simulink model "Model_with_decision"  (R2022a)
settings: Solver=VariableStepAuto  StartTime=0.0  StopTime=1000000  RelTol=1e-3
undefined symbols (not defined in the file): Coefficient_value, Enable_X, Enable_Y, N, s1, s10, s11, s12, s13, s14, s15, s16, s17, s18, s19, s2, s20, s21, s22, s23, s24, s25, s26, s27, s28, s29, s3, s30, s4, s5, s6, s7, s8, s9
libraries: simulink x35
(part 3 of 5)

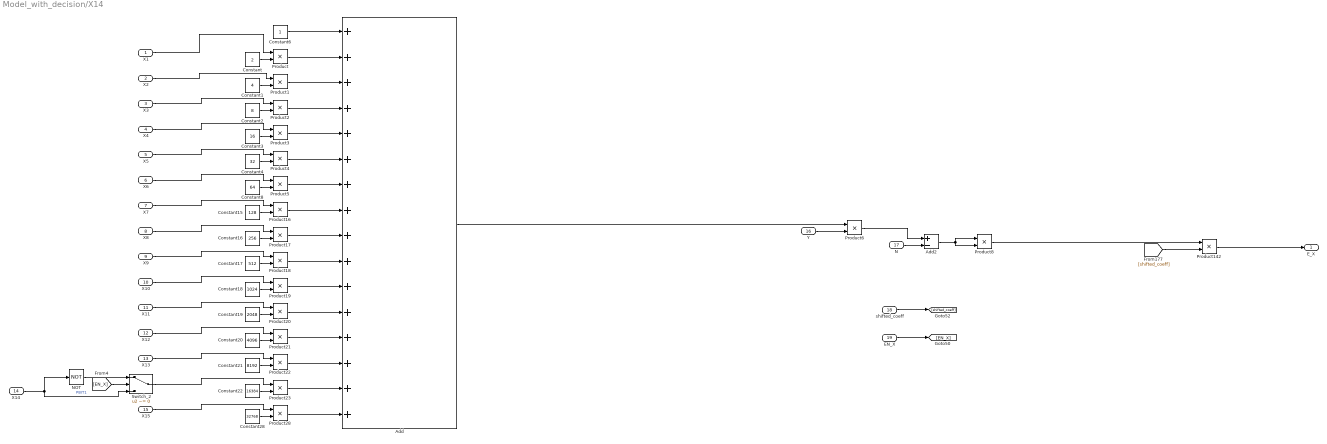
== system Model_with_decision/X14 ==
  X1 : Inport  OutDataTypeStr=fixdt(0,1,0)  LockScale=on
  X2 : Inport  Port=2  OutDataTypeStr=fixdt(0,1,0)  LockScale=on
  X3 : Inport  Port=3  OutDataTypeStr=fixdt(0,1,0)  LockScale=on
  X4 : Inport  Port=4  OutDataTypeStr=fixdt(0,1,0)  LockScale=on
  X5 : Inport  Port=5  OutDataTypeStr=fixdt(0,1,0)  LockScale=on
  X6 : Inport  Port=6  OutDataTypeStr=fixdt(0,1,0)  LockScale=on
  X7 : Inport  Port=7  OutDataTypeStr=fixdt(0,1,0)  LockScale=on
  X8 : Inport  Port=8  OutDataTypeStr=fixdt(0,1,0)  LockScale=on
  X9 : Inport  Port=9  OutDataTypeStr=fixdt(0,1,0)  LockScale=on
  X10 : Inport  Port=10  OutDataTypeStr=fixdt(0,1,0)  LockScale=on
  X11 : Inport  Port=11  OutDataTypeStr=fixdt(0,1,0)  LockScale=on
  X12 : Inport  Port=12  OutDataTypeStr=fixdt(0,1,0)  LockScale=on
  X13 : Inport  Port=13  OutDataTypeStr=fixdt(0,1,0)  LockScale=on
  X14 : Inport  Port=14  OutDataTypeStr=fixdt(0,1,0)  LockScale=on
  X15 : Inport  Port=15  OutDataTypeStr=fixdt(0,1,0)  LockScale=on
  Y : Inport  Port=16  LockScale=on
  N : Inport  Port=17  LockScale=on
  shifted_coeff : Inport  Port=18  LockScale=on
  EN_X : Inport  Port=19  OutDataTypeStr=fixdt(0,1,0)  LockScale=on
  Add : Sum  Inputs=++++++++++++++++
  Add2 : Sum  Inputs=+-
  Constant : Constant  Value=2
  Constant1 : Constant  Value=4
  Constant15 : Constant  Value=128
  Constant16 : Constant  Value=256
  Constant17 : Constant  Value=512
  Constant18 : Constant  Value=1024
  Constant19 : Constant  Value=2048
  Constant2 : Constant  Value=8
  Constant20 : Constant  Value=4096
  Constant21 : Constant  Value=8192
  Constant22 : Constant  Value=16384
  Constant28 : Constant  Value=32768
  Constant3 : Constant  Value=16
  Constant4 : Constant  Value=32
  Constant6 : Constant
  Constant8 : Constant  Value=64
  NOT : Logic  Operator=NOT  IconShape=distinctive  AllPortsSameDT=off  OutDataTypeStr=boolean
  Product{,1..6,8,16..23,28,142} (18 alike) : Product
  Switch_2 : Switch  Criteria=u2 ~= 0  OutDataTypeStr=fixdt(0,1,0)  SaturateOnIntegerOverflow=off  InputSameDT=off
  E_X : Outport  LockScale=on
  wires:
  Y/1 -> Product6/2
  N/1 -> Add2/2
  Product8/1 -> Product142/1
  Product6/1 -> Add2/1
  [shifted_coeff] -> Product142/2
  Product142/1 -> E_X/1
  shifted_coeff/1 -> [shifted_coeff]
  EN_X/1 -> [EN_X]
  X13/1 -> Product22/1
  NOT/1 -> Switch_2/1
  X14/1 -> NOT/1, Switch_2/3  "PBIT1"
  [EN_X] -> Switch_2/2
  Constant22/1 -> Product23/2
  Constant21/1 -> Product22/2
  Product23/1 -> Add/15
  Product22/1 -> Add/14
  Product28/1 -> Add/16
  Constant28/1 -> Product28/2
  X15/1 -> Product28/1
  Switch_2/1 -> Product23/1
  Product17/1 -> Add/9
  X12/1 -> Product21/1
  Product21/1 -> Add/13
  Constant17/1 -> Product18/2
  X9/1 -> Product18/1
  Product16/1 -> Add/8
  Constant19/1 -> Product20/2
  X7/1 -> Product16/1
  X10/1 -> Product19/1
  X8/1 -> Product17/1
  Product20/1 -> Add/12
  X11/1 -> Product20/1
  Constant16/1 -> Product17/2
  Constant15/1 -> Product16/2
  Product18/1 -> Add/10
  Constant18/1 -> Product19/2
  Constant20/1 -> Product21/2
  Product19/1 -> Add/11
  Constant3/1 -> Product3/2
  X5/1 -> Product4/1
  Product5/1 -> Add/7
  X4/1 -> Product3/1
  Product3/1 -> Add/5
  X6/1 -> Product5/1
  Constant8/1 -> Product5/2
  Constant4/1 -> Product4/2
  Product4/1 -> Add/6
  Add2/1 -> Product8/1, Product8/2
  Add/1 -> Product6/1
  Product2/1 -> Add/4
  Product1/1 -> Add/3
  Product/1 -> Add/2
  Constant6/1 -> Add/1
  X3/1 -> Product2/1
  Constant2/1 -> Product2/2
  X2/1 -> Product1/1
  Constant1/1 -> Product1/2
  X1/1 -> Product/1
  Constant/1 -> Product/2

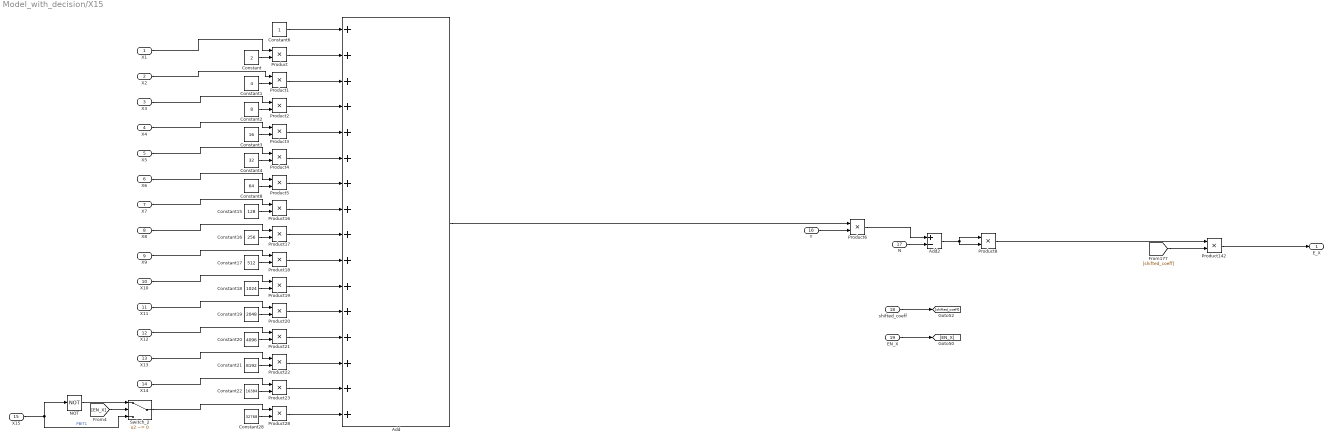
== system Model_with_decision/X15 ==
  X1 : Inport  OutDataTypeStr=fixdt(0,1,0)  LockScale=on
  X2 : Inport  Port=2  OutDataTypeStr=fixdt(0,1,0)  LockScale=on
  X3 : Inport  Port=3  OutDataTypeStr=fixdt(0,1,0)  LockScale=on
  X4 : Inport  Port=4  OutDataTypeStr=fixdt(0,1,0)  LockScale=on
  X5 : Inport  Port=5  OutDataTypeStr=fixdt(0,1,0)  LockScale=on
  X6 : Inport  Port=6  OutDataTypeStr=fixdt(0,1,0)  LockScale=on
  X7 : Inport  Port=7  OutDataTypeStr=fixdt(0,1,0)  LockScale=on
  X8 : Inport  Port=8  OutDataTypeStr=fixdt(0,1,0)  LockScale=on
  X9 : Inport  Port=9  OutDataTypeStr=fixdt(0,1,0)  LockScale=on
  X10 : Inport  Port=10  OutDataTypeStr=fixdt(0,1,0)  LockScale=on
  X11 : Inport  Port=11  OutDataTypeStr=fixdt(0,1,0)  LockScale=on
  X12 : Inport  Port=12  OutDataTypeStr=fixdt(0,1,0)  LockScale=on
  X13 : Inport  Port=13  OutDataTypeStr=fixdt(0,1,0)  LockScale=on
  X14 : Inport  Port=14  OutDataTypeStr=fixdt(0,1,0)  LockScale=on
  X15 : Inport  Port=15  OutDataTypeStr=fixdt(0,1,0)  LockScale=on
  Y : Inport  Port=16  LockScale=on
  N : Inport  Port=17  LockScale=on
  shifted_coeff : Inport  Port=18  LockScale=on
  EN_X : Inport  Port=19  OutDataTypeStr=fixdt(0,1,0)  LockScale=on
  Add : Sum  Inputs=++++++++++++++++
  Add2 : Sum  Inputs=+-
  Constant : Constant  Value=2
  Constant1 : Constant  Value=4
  Constant15 : Constant  Value=128
  Constant16 : Constant  Value=256
  Constant17 : Constant  Value=512
  Constant18 : Constant  Value=1024
  Constant19 : Constant  Value=2048
  Constant2 : Constant  Value=8
  Constant20 : Constant  Value=4096
  Constant21 : Constant  Value=8192
  Constant22 : Constant  Value=16384
  Constant28 : Constant  Value=32768
  Constant3 : Constant  Value=16
  Constant4 : Constant  Value=32
  Constant6 : Constant
  Constant8 : Constant  Value=64
  NOT : Logic  Operator=NOT  IconShape=distinctive  AllPortsSameDT=off  OutDataTypeStr=boolean
  Product{,1..6,8,16..23,28,142} (18 alike) : Product
  Switch_2 : Switch  Criteria=u2 ~= 0  OutDataTypeStr=fixdt(0,1,0)  SaturateOnIntegerOverflow=off  InputSameDT=off
  E_X : Outport  LockScale=on
  wires:
  Constant/1 -> Product/2
  X1/1 -> Product/1
  Constant1/1 -> Product1/2
  X2/1 -> Product1/1
  Constant2/1 -> Product2/2
  X3/1 -> Product2/1
  Constant6/1 -> Add/1
  Product/1 -> Add/2
  Product1/1 -> Add/3
  Product2/1 -> Add/4
  Add/1 -> Product6/1
  Add2/1 -> Product8/2, Product8/1
  Product4/1 -> Add/6
  Constant4/1 -> Product4/2
  Constant8/1 -> Product5/2
  X6/1 -> Product5/1
  Product3/1 -> Add/5
  X4/1 -> Product3/1
  Product5/1 -> Add/7
  X5/1 -> Product4/1
  Constant3/1 -> Product3/2
  Product19/1 -> Add/11
  Constant20/1 -> Product21/2
  Constant18/1 -> Product19/2
  Product18/1 -> Add/10
  Constant15/1 -> Product16/2
  Constant16/1 -> Product17/2
  X11/1 -> Product20/1
  Product20/1 -> Add/12
  X8/1 -> Product17/1
  X10/1 -> Product19/1
  X7/1 -> Product16/1
  Constant19/1 -> Product20/2
  Product16/1 -> Add/8
  X9/1 -> Product18/1
  Constant17/1 -> Product18/2
  Product21/1 -> Add/13
  X12/1 -> Product21/1
  Product17/1 -> Add/9
  X14/1 -> Product23/1
  Switch_2/1 -> Product28/1
  Constant28/1 -> Product28/2
  Product28/1 -> Add/16
  Product22/1 -> Add/14
  Product23/1 -> Add/15
  Constant21/1 -> Product22/2
  Constant22/1 -> Product23/2
  [EN_X] -> Switch_2/2
  X15/1 -> Switch_2/3, NOT/1  "PBIT1"
  NOT/1 -> Switch_2/1
  X13/1 -> Product22/1
  EN_X/1 -> [EN_X]
  shifted_coeff/1 -> [shifted_coeff]
  Product142/1 -> E_X/1
  [shifted_coeff] -> Product142/2
  Product6/1 -> Add2/1
  Product8/1 -> Product142/1
  N/1 -> Add2/2
  Y/1 -> Product6/2

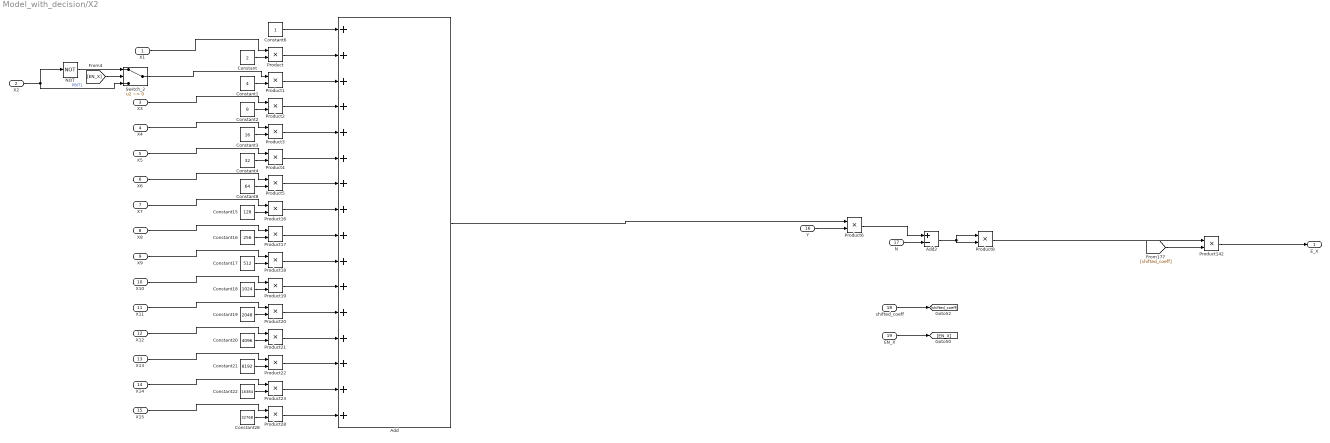
== system Model_with_decision/X2 ==
  X1 : Inport  OutDataTypeStr=fixdt(0,1,0)  LockScale=on
  X2 : Inport  Port=2  OutDataTypeStr=fixdt(0,1,0)  LockScale=on
  X3 : Inport  Port=3  OutDataTypeStr=fixdt(0,1,0)  LockScale=on
  X4 : Inport  Port=4  OutDataTypeStr=fixdt(0,1,0)  LockScale=on
  X5 : Inport  Port=5  OutDataTypeStr=fixdt(0,1,0)  LockScale=on
  X6 : Inport  Port=6  OutDataTypeStr=fixdt(0,1,0)  LockScale=on
  X7 : Inport  Port=7  OutDataTypeStr=fixdt(0,1,0)  LockScale=on
  X8 : Inport  Port=8  OutDataTypeStr=fixdt(0,1,0)  LockScale=on
  X9 : Inport  Port=9  OutDataTypeStr=fixdt(0,1,0)  LockScale=on
  X10 : Inport  Port=10  OutDataTypeStr=fixdt(0,1,0)  LockScale=on
  X11 : Inport  Port=11  OutDataTypeStr=fixdt(0,1,0)  LockScale=on
  X12 : Inport  Port=12  OutDataTypeStr=fixdt(0,1,0)  LockScale=on
  X13 : Inport  Port=13  OutDataTypeStr=fixdt(0,1,0)  LockScale=on
  X14 : Inport  Port=14  OutDataTypeStr=fixdt(0,1,0)  LockScale=on
  X15 : Inport  Port=15  OutDataTypeStr=fixdt(0,1,0)  LockScale=on
  Y : Inport  Port=16  LockScale=on
  N : Inport  Port=17  LockScale=on
  shifted_coeff : Inport  Port=18  LockScale=on
  EN_X : Inport  Port=19  OutDataTypeStr=fixdt(0,1,0)  LockScale=on
  Add : Sum  Inputs=++++++++++++++++
  Add2 : Sum  Inputs=+-
  Constant : Constant  Value=2
  Constant1 : Constant  Value=4
  Constant15 : Constant  Value=128
  Constant16 : Constant  Value=256
  Constant17 : Constant  Value=512
  Constant18 : Constant  Value=1024
  Constant19 : Constant  Value=2048
  Constant2 : Constant  Value=8
  Constant20 : Constant  Value=4096
  Constant21 : Constant  Value=8192
  Constant22 : Constant  Value=16384
  Constant28 : Constant  Value=32768
  Constant3 : Constant  Value=16
  Constant4 : Constant  Value=32
  Constant6 : Constant
  Constant8 : Constant  Value=64
  NOT : Logic  Operator=NOT  IconShape=distinctive  AllPortsSameDT=off  OutDataTypeStr=boolean
  Product{,1..6,8,16..23,28,142} (18 alike) : Product
  Switch_2 : Switch  Criteria=u2 ~= 0  OutDataTypeStr=fixdt(0,1,0)  SaturateOnIntegerOverflow=off  InputSameDT=off
  E_X : Outport  LockScale=on
  wires:
  Y/1 -> Product6/2
  N/1 -> Add2/2
  Product8/1 -> Product142/1
  Product6/1 -> Add2/1
  [shifted_coeff] -> Product142/2
  Product142/1 -> E_X/1
  shifted_coeff/1 -> [shifted_coeff]
  EN_X/1 -> [EN_X]
  X13/1 -> Product22/1
  NOT/1 -> Switch_2/1
  X2/1 -> Switch_2/3, NOT/1  "PBIT1"
  [EN_X] -> Switch_2/2
  Constant22/1 -> Product23/2
  Constant21/1 -> Product22/2
  Product23/1 -> Add/15
  Product22/1 -> Add/14
  Product28/1 -> Add/16
  Constant28/1 -> Product28/2
  X15/1 -> Product28/1
  X14/1 -> Product23/1
  Product17/1 -> Add/9
  X12/1 -> Product21/1
  Product21/1 -> Add/13
  Constant17/1 -> Product18/2
  X9/1 -> Product18/1
  Product16/1 -> Add/8
  Constant19/1 -> Product20/2
  X7/1 -> Product16/1
  X10/1 -> Product19/1
  X8/1 -> Product17/1
  Product20/1 -> Add/12
  X11/1 -> Product20/1
  Constant16/1 -> Product17/2
  Constant15/1 -> Product16/2
  Product18/1 -> Add/10
  Constant18/1 -> Product19/2
  Constant20/1 -> Product21/2
  Product19/1 -> Add/11
  Constant3/1 -> Product3/2
  X5/1 -> Product4/1
  Product5/1 -> Add/7
  X4/1 -> Product3/1
  Product3/1 -> Add/5
  X6/1 -> Product5/1
  Constant8/1 -> Product5/2
  Constant4/1 -> Product4/2
  Product4/1 -> Add/6
  Add2/1 -> Product8/1, Product8/2
  Add/1 -> Product6/1
  Product2/1 -> Add/4
  Product1/1 -> Add/3
  Product/1 -> Add/2
  Constant6/1 -> Add/1
  X3/1 -> Product2/1
  Constant2/1 -> Product2/2
  Switch_2/1 -> Product1/1
  Constant1/1 -> Product1/2
  X1/1 -> Product/1
  Constant/1 -> Product/2

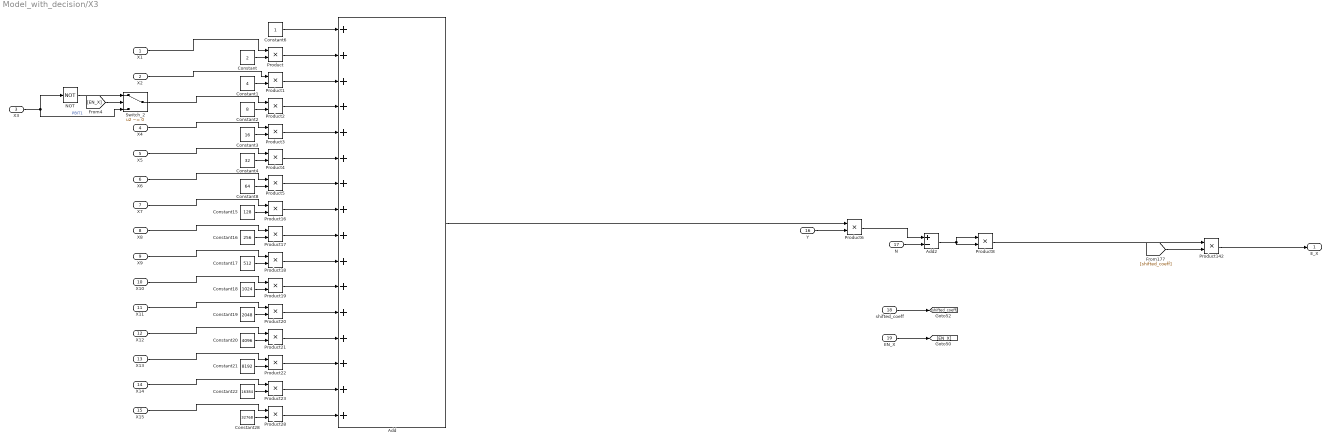
== system Model_with_decision/X3 ==
  X1 : Inport  OutDataTypeStr=fixdt(0,1,0)  LockScale=on
  X2 : Inport  Port=2  OutDataTypeStr=fixdt(0,1,0)  LockScale=on
  X3 : Inport  Port=3  OutDataTypeStr=fixdt(0,1,0)  LockScale=on
  X4 : Inport  Port=4  OutDataTypeStr=fixdt(0,1,0)  LockScale=on
  X5 : Inport  Port=5  OutDataTypeStr=fixdt(0,1,0)  LockScale=on
  X6 : Inport  Port=6  OutDataTypeStr=fixdt(0,1,0)  LockScale=on
  X7 : Inport  Port=7  OutDataTypeStr=fixdt(0,1,0)  LockScale=on
  X8 : Inport  Port=8  OutDataTypeStr=fixdt(0,1,0)  LockScale=on
  X9 : Inport  Port=9  OutDataTypeStr=fixdt(0,1,0)  LockScale=on
  X10 : Inport  Port=10  OutDataTypeStr=fixdt(0,1,0)  LockScale=on
  X11 : Inport  Port=11  OutDataTypeStr=fixdt(0,1,0)  LockScale=on
  X12 : Inport  Port=12  OutDataTypeStr=fixdt(0,1,0)  LockScale=on
  X13 : Inport  Port=13  OutDataTypeStr=fixdt(0,1,0)  LockScale=on
  X14 : Inport  Port=14  OutDataTypeStr=fixdt(0,1,0)  LockScale=on
  X15 : Inport  Port=15  OutDataTypeStr=fixdt(0,1,0)  LockScale=on
  Y : Inport  Port=16  LockScale=on
  N : Inport  Port=17  LockScale=on
  shifted_coeff : Inport  Port=18  LockScale=on
  EN_X : Inport  Port=19  OutDataTypeStr=fixdt(0,1,0)  LockScale=on
  Add : Sum  Inputs=++++++++++++++++
  Add2 : Sum  Inputs=+-
  Constant : Constant  Value=2
  Constant1 : Constant  Value=4
  Constant15 : Constant  Value=128
  Constant16 : Constant  Value=256
  Constant17 : Constant  Value=512
  Constant18 : Constant  Value=1024
  Constant19 : Constant  Value=2048
  Constant2 : Constant  Value=8
  Constant20 : Constant  Value=4096
  Constant21 : Constant  Value=8192
  Constant22 : Constant  Value=16384
  Constant28 : Constant  Value=32768
  Constant3 : Constant  Value=16
  Constant4 : Constant  Value=32
  Constant6 : Constant
  Constant8 : Constant  Value=64
  NOT : Logic  Operator=NOT  IconShape=distinctive  AllPortsSameDT=off  OutDataTypeStr=boolean
  Product{,1..6,8,16..23,28,142} (18 alike) : Product
  Switch_2 : Switch  Criteria=u2 ~= 0  OutDataTypeStr=fixdt(0,1,0)  SaturateOnIntegerOverflow=off  InputSameDT=off
  E_X : Outport  LockScale=on
  wires:
  Y/1 -> Product6/2
  N/1 -> Add2/2
  Product8/1 -> Product142/1
  Product6/1 -> Add2/1
  [shifted_coeff] -> Product142/2
  Product142/1 -> E_X/1
  shifted_coeff/1 -> [shifted_coeff]
  EN_X/1 -> [EN_X]
  X13/1 -> Product22/1
  NOT/1 -> Switch_2/1
  X3/1 -> Switch_2/3, NOT/1  "PBIT1"
  [EN_X] -> Switch_2/2
  Constant22/1 -> Product23/2
  Constant21/1 -> Product22/2
  Product23/1 -> Add/15
  Product22/1 -> Add/14
  Product28/1 -> Add/16
  Constant28/1 -> Product28/2
  X15/1 -> Product28/1
  X14/1 -> Product23/1
  Product17/1 -> Add/9
  X12/1 -> Product21/1
  Product21/1 -> Add/13
  Constant17/1 -> Product18/2
  X9/1 -> Product18/1
  Product16/1 -> Add/8
  Constant19/1 -> Product20/2
  X7/1 -> Product16/1
  X10/1 -> Product19/1
  X8/1 -> Product17/1
  Product20/1 -> Add/12
  X11/1 -> Product20/1
  Constant16/1 -> Product17/2
  Constant15/1 -> Product16/2
  Product18/1 -> Add/10
  Constant18/1 -> Product19/2
  Constant20/1 -> Product21/2
  Product19/1 -> Add/11
  Constant3/1 -> Product3/2
  X5/1 -> Product4/1
  Product5/1 -> Add/7
  X4/1 -> Product3/1
  Product3/1 -> Add/5
  X6/1 -> Product5/1
  Constant8/1 -> Product5/2
  Constant4/1 -> Product4/2
  Product4/1 -> Add/6
  Add2/1 -> Product8/1, Product8/2
  Add/1 -> Product6/1
  Product2/1 -> Add/4
  Product1/1 -> Add/3
  Product/1 -> Add/2
  Constant6/1 -> Add/1
  Switch_2/1 -> Product2/1
  Constant2/1 -> Product2/2
  X2/1 -> Product1/1
  Constant1/1 -> Product1/2
  X1/1 -> Product/1
  Constant/1 -> Product/2

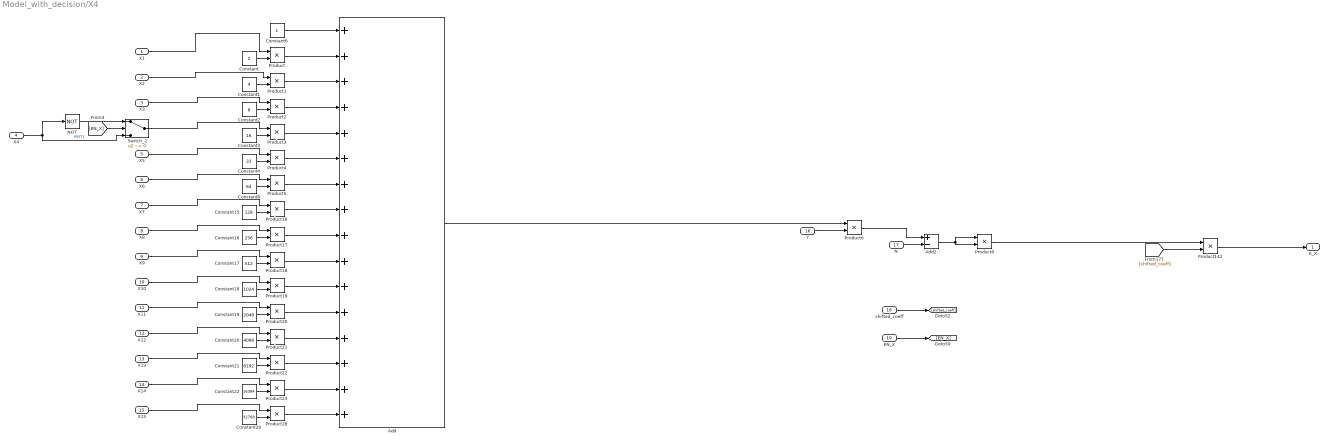
== system Model_with_decision/X4 ==
  X1 : Inport  OutDataTypeStr=fixdt(0,1,0)  LockScale=on
  X2 : Inport  Port=2  OutDataTypeStr=fixdt(0,1,0)  LockScale=on
  X3 : Inport  Port=3  OutDataTypeStr=fixdt(0,1,0)  LockScale=on
  X4 : Inport  Port=4  OutDataTypeStr=fixdt(0,1,0)  LockScale=on
  X5 : Inport  Port=5  OutDataTypeStr=fixdt(0,1,0)  LockScale=on
  X6 : Inport  Port=6  OutDataTypeStr=fixdt(0,1,0)  LockScale=on
  X7 : Inport  Port=7  OutDataTypeStr=fixdt(0,1,0)  LockScale=on
  X8 : Inport  Port=8  OutDataTypeStr=fixdt(0,1,0)  LockScale=on
  X9 : Inport  Port=9  OutDataTypeStr=fixdt(0,1,0)  LockScale=on
  X10 : Inport  Port=10  OutDataTypeStr=fixdt(0,1,0)  LockScale=on
  X11 : Inport  Port=11  OutDataTypeStr=fixdt(0,1,0)  LockScale=on
  X12 : Inport  Port=12  OutDataTypeStr=fixdt(0,1,0)  LockScale=on
  X13 : Inport  Port=13  OutDataTypeStr=fixdt(0,1,0)  LockScale=on
  X14 : Inport  Port=14  OutDataTypeStr=fixdt(0,1,0)  LockScale=on
  X15 : Inport  Port=15  OutDataTypeStr=fixdt(0,1,0)  LockScale=on
  Y : Inport  Port=16  LockScale=on
  N : Inport  Port=17  LockScale=on
  shifted_coeff : Inport  Port=18  LockScale=on
  EN_X : Inport  Port=19  OutDataTypeStr=fixdt(0,1,0)  LockScale=on
  Add : Sum  Inputs=++++++++++++++++
  Add2 : Sum  Inputs=+-
  Constant : Constant  Value=2
  Constant1 : Constant  Value=4
  Constant15 : Constant  Value=128
  Constant16 : Constant  Value=256
  Constant17 : Constant  Value=512
  Constant18 : Constant  Value=1024
  Constant19 : Constant  Value=2048
  Constant2 : Constant  Value=8
  Constant20 : Constant  Value=4096
  Constant21 : Constant  Value=8192
  Constant22 : Constant  Value=16384
  Constant28 : Constant  Value=32768
  Constant3 : Constant  Value=16
  Constant4 : Constant  Value=32
  Constant6 : Constant
  Constant8 : Constant  Value=64
  NOT : Logic  Operator=NOT  IconShape=distinctive  AllPortsSameDT=off  OutDataTypeStr=boolean
  Product{,1..6,8,16..23,28,142} (18 alike) : Product
  Switch_2 : Switch  Criteria=u2 ~= 0  OutDataTypeStr=fixdt(0,1,0)  SaturateOnIntegerOverflow=off  InputSameDT=off
  E_X : Outport  LockScale=on
  wires:
  Constant/1 -> Product/2
  X1/1 -> Product/1
  Constant1/1 -> Product1/2
  X2/1 -> Product1/1
  Constant2/1 -> Product2/2
  X3/1 -> Product2/1
  Constant6/1 -> Add/1
  Product/1 -> Add/2
  Product1/1 -> Add/3
  Product2/1 -> Add/4
  Add/1 -> Product6/1
  Add2/1 -> Product8/2, Product8/1
  Product4/1 -> Add/6
  Constant4/1 -> Product4/2
  Constant8/1 -> Product5/2
  X6/1 -> Product5/1
  Product3/1 -> Add/5
  Switch_2/1 -> Product3/1
  Product5/1 -> Add/7
  X5/1 -> Product4/1
  Constant3/1 -> Product3/2
  Product19/1 -> Add/11
  Constant20/1 -> Product21/2
  Constant18/1 -> Product19/2
  Product18/1 -> Add/10
  Constant15/1 -> Product16/2
  Constant16/1 -> Product17/2
  X11/1 -> Product20/1
  Product20/1 -> Add/12
  X8/1 -> Product17/1
  X10/1 -> Product19/1
  X7/1 -> Product16/1
  Constant19/1 -> Product20/2
  Product16/1 -> Add/8
  X9/1 -> Product18/1
  Constant17/1 -> Product18/2
  Product21/1 -> Add/13
  X12/1 -> Product21/1
  Product17/1 -> Add/9
  X14/1 -> Product23/1
  X15/1 -> Product28/1
  Constant28/1 -> Product28/2
  Product28/1 -> Add/16
  Product22/1 -> Add/14
  Product23/1 -> Add/15
  Constant21/1 -> Product22/2
  Constant22/1 -> Product23/2
  [EN_X] -> Switch_2/2
  X4/1 -> NOT/1, Switch_2/3  "PBIT1"
  NOT/1 -> Switch_2/1
  X13/1 -> Product22/1
  EN_X/1 -> [EN_X]
  shifted_coeff/1 -> [shifted_coeff]
  Product142/1 -> E_X/1
  [shifted_coeff] -> Product142/2
  Product6/1 -> Add2/1
  Product8/1 -> Product142/1
  N/1 -> Add2/2
  Y/1 -> Product6/2

== system Model_with_decision/X5 ==
  X1 : Inport  OutDataTypeStr=fixdt(0,1,0)  LockScale=on
  X2 : Inport  Port=2  OutDataTypeStr=fixdt(0,1,0)  LockScale=on
  X3 : Inport  Port=3  OutDataTypeStr=fixdt(0,1,0)  LockScale=on
  X4 : Inport  Port=4  OutDataTypeStr=fixdt(0,1,0)  LockScale=on
  X5 : Inport  Port=5  OutDataTypeStr=fixdt(0,1,0)  LockScale=on
  X6 : Inport  Port=6  OutDataTypeStr=fixdt(0,1,0)  LockScale=on
  X7 : Inport  Port=7  OutDataTypeStr=fixdt(0,1,0)  LockScale=on
  X8 : Inport  Port=8  OutDataTypeStr=fixdt(0,1,0)  LockScale=on
  X9 : Inport  Port=9  OutDataTypeStr=fixdt(0,1,0)  LockScale=on
  X10 : Inport  Port=10  OutDataTypeStr=fixdt(0,1,0)  LockScale=on
  X11 : Inport  Port=11  OutDataTypeStr=fixdt(0,1,0)  LockScale=on
  X12 : Inport  Port=12  OutDataTypeStr=fixdt(0,1,0)  LockScale=on
  X13 : Inport  Port=13  OutDataTypeStr=fixdt(0,1,0)  LockScale=on
  X14 : Inport  Port=14  OutDataTypeStr=fixdt(0,1,0)  LockScale=on
  X15 : Inport  Port=15  OutDataTypeStr=fixdt(0,1,0)  LockScale=on
  Y : Inport  Port=16  LockScale=on
  N : Inport  Port=17  LockScale=on
  shifted_coeff : Inport  Port=18  LockScale=on
  EN_X : Inport  Port=19  OutDataTypeStr=fixdt(0,1,0)  LockScale=on
  Add : Sum  Inputs=++++++++++++++++
  Add2 : Sum  Inputs=+-
  Constant : Constant  Value=2
  Constant1 : Constant  Value=4
  Constant15 : Constant  Value=128
  Constant16 : Constant  Value=256
  Constant17 : Constant  Value=512
  Constant18 : Constant  Value=1024
  Constant19 : Constant  Value=2048
  Constant2 : Constant  Value=8
  Constant20 : Constant  Value=4096
  Constant21 : Constant  Value=8192
  Constant22 : Constant  Value=16384
  Constant28 : Constant  Value=32768
  Constant3 : Constant  Value=16
  Constant4 : Constant  Value=32
  Constant6 : Constant
  Constant8 : Constant  Value=64
  NOT : Logic  Operator=NOT  IconShape=distinctive  AllPortsSameDT=off  OutDataTypeStr=boolean
  Product{,1..6,8,16..23,28,142} (18 alike) : Product
  Switch_2 : Switch  Criteria=u2 ~= 0  OutDataTypeStr=fixdt(0,1,0)  SaturateOnIntegerOverflow=off  InputSameDT=off
  E_X : Outport  LockScale=on
  wires:
  Y/1 -> Product6/2
  N/1 -> Add2/2
  Product8/1 -> Product142/1
  Product6/1 -> Add2/1
  [shifted_coeff] -> Product142/2
  Product142/1 -> E_X/1
  shifted_coeff/1 -> [shifted_coeff]
  EN_X/1 -> [EN_X]
  X13/1 -> Product22/1
  NOT/1 -> Switch_2/1
  X5/1 -> NOT/1, Switch_2/3  "PBIT1"
  [EN_X] -> Switch_2/2
  Constant22/1 -> Product23/2
  Constant21/1 -> Product22/2
  Product23/1 -> Add/15
  Product22/1 -> Add/14
  Product28/1 -> Add/16
  Constant28/1 -> Product28/2
  X15/1 -> Product28/1
  X14/1 -> Product23/1
  Product17/1 -> Add/9
  X12/1 -> Product21/1
  Product21/1 -> Add/13
  Constant17/1 -> Product18/2
  X9/1 -> Product18/1
  Product16/1 -> Add/8
  Constant19/1 -> Product20/2
  X7/1 -> Product16/1
  X10/1 -> Product19/1
  X8/1 -> Product17/1
  Product20/1 -> Add/12
  X11/1 -> Product20/1
  Constant16/1 -> Product17/2
  Constant15/1 -> Product16/2
  Product18/1 -> Add/10
  Constant18/1 -> Product19/2
  Constant20/1 -> Product21/2
  Product19/1 -> Add/11
  Constant3/1 -> Product3/2
  Switch_2/1 -> Product4/1
  Product5/1 -> Add/7
  X4/1 -> Product3/1
  Product3/1 -> Add/5
  X6/1 -> Product5/1
  Constant8/1 -> Product5/2
  Constant4/1 -> Product4/2
  Product4/1 -> Add/6
  Add2/1 -> Product8/1, Product8/2
  Add/1 -> Product6/1
  Product2/1 -> Add/4
  Product1/1 -> Add/3
  Product/1 -> Add/2
  Constant6/1 -> Add/1
  X3/1 -> Product2/1
  Constant2/1 -> Product2/2
  X2/1 -> Product1/1
  Constant1/1 -> Product1/2
  X1/1 -> Product/1
  Constant/1 -> Product/2

== system Model_with_decision/X6 ==
  X1 : Inport  OutDataTypeStr=fixdt(0,1,0)  LockScale=on
  X2 : Inport  Port=2  OutDataTypeStr=fixdt(0,1,0)  LockScale=on
  X3 : Inport  Port=3  OutDataTypeStr=fixdt(0,1,0)  LockScale=on
  X4 : Inport  Port=4  OutDataTypeStr=fixdt(0,1,0)  LockScale=on
  X5 : Inport  Port=5  OutDataTypeStr=fixdt(0,1,0)  LockScale=on
  X6 : Inport  Port=6  OutDataTypeStr=fixdt(0,1,0)  LockScale=on
  X7 : Inport  Port=7  OutDataTypeStr=fixdt(0,1,0)  LockScale=on
  X8 : Inport  Port=8  OutDataTypeStr=fixdt(0,1,0)  LockScale=on
  X9 : Inport  Port=9  OutDataTypeStr=fixdt(0,1,0)  LockScale=on
  X10 : Inport  Port=10  OutDataTypeStr=fixdt(0,1,0)  LockScale=on
  X11 : Inport  Port=11  OutDataTypeStr=fixdt(0,1,0)  LockScale=on
  X12 : Inport  Port=12  OutDataTypeStr=fixdt(0,1,0)  LockScale=on
  X13 : Inport  Port=13  OutDataTypeStr=fixdt(0,1,0)  LockScale=on
  X14 : Inport  Port=14  OutDataTypeStr=fixdt(0,1,0)  LockScale=on
  X15 : Inport  Port=15  OutDataTypeStr=fixdt(0,1,0)  LockScale=on
  Y : Inport  Port=16  LockScale=on
  N : Inport  Port=17  LockScale=on
  shifted_coeff : Inport  Port=18  LockScale=on
  EN_X : Inport  Port=19  OutDataTypeStr=fixdt(0,1,0)  LockScale=on
  Add : Sum  Inputs=++++++++++++++++
  Add2 : Sum  Inputs=+-
  Constant : Constant  Value=2
  Constant1 : Constant  Value=4
  Constant15 : Constant  Value=128
  Constant16 : Constant  Value=256
  Constant17 : Constant  Value=512
  Constant18 : Constant  Value=1024
  Constant19 : Constant  Value=2048
  Constant2 : Constant  Value=8
  Constant20 : Constant  Value=4096
  Constant21 : Constant  Value=8192
  Constant22 : Constant  Value=16384
  Constant28 : Constant  Value=32768
  Constant3 : Constant  Value=16
  Constant4 : Constant  Value=32
  Constant6 : Constant
  Constant8 : Constant  Value=64
  NOT : Logic  Operator=NOT  IconShape=distinctive  AllPortsSameDT=off  OutDataTypeStr=boolean
  Product{,1..6,8,16..23,28,142} (18 alike) : Product
  Switch_2 : Switch  Criteria=u2 ~= 0  OutDataTypeStr=fixdt(0,1,0)  SaturateOnIntegerOverflow=off  InputSameDT=off
  E_X : Outport  LockScale=on
  wires:
  Y/1 -> Product6/2
  N/1 -> Add2/2
  Product8/1 -> Product142/1
  Product6/1 -> Add2/1
  [shifted_coeff] -> Product142/2
  Product142/1 -> E_X/1
  shifted_coeff/1 -> [shifted_coeff]
  EN_X/1 -> [EN_X]
  X13/1 -> Product22/1
  NOT/1 -> Switch_2/1
  X6/1 -> NOT/1, Switch_2/3  "PBIT1"
  [EN_X] -> Switch_2/2
  Constant22/1 -> Product23/2
  Constant21/1 -> Product22/2
  Product23/1 -> Add/15
  Product22/1 -> Add/14
  Product28/1 -> Add/16
  Constant28/1 -> Product28/2
  X15/1 -> Product28/1
  X14/1 -> Product23/1
  Product17/1 -> Add/9
  X12/1 -> Product21/1
  Product21/1 -> Add/13
  Constant17/1 -> Product18/2
  X9/1 -> Product18/1
  Product16/1 -> Add/8
  Constant19/1 -> Product20/2
  X7/1 -> Product16/1
  X10/1 -> Product19/1
  X8/1 -> Product17/1
  Product20/1 -> Add/12
  X11/1 -> Product20/1
  Constant16/1 -> Product17/2
  Constant15/1 -> Product16/2
  Product18/1 -> Add/10
  Constant18/1 -> Product19/2
  Constant20/1 -> Product21/2
  Product19/1 -> Add/11
  Constant3/1 -> Product3/2
  X5/1 -> Product4/1
  Product5/1 -> Add/7
  X4/1 -> Product3/1
  Product3/1 -> Add/5
  Switch_2/1 -> Product5/1
  Constant8/1 -> Product5/2
  Constant4/1 -> Product4/2
  Product4/1 -> Add/6
  Add2/1 -> Product8/1, Product8/2
  Add/1 -> Product6/1
  Product2/1 -> Add/4
  Product1/1 -> Add/3
  Product/1 -> Add/2
  Constant6/1 -> Add/1
  X3/1 -> Product2/1
  Constant2/1 -> Product2/2
  X2/1 -> Product1/1
  Constant1/1 -> Product1/2
  X1/1 -> Product/1
  Constant/1 -> Product/2

== system Model_with_decision/X7 ==
  X1 : Inport  OutDataTypeStr=fixdt(0,1,0)  LockScale=on
  X2 : Inport  Port=2  OutDataTypeStr=fixdt(0,1,0)  LockScale=on
  X3 : Inport  Port=3  OutDataTypeStr=fixdt(0,1,0)  LockScale=on
  X4 : Inport  Port=4  OutDataTypeStr=fixdt(0,1,0)  LockScale=on
  X5 : Inport  Port=5  OutDataTypeStr=fixdt(0,1,0)  LockScale=on
  X6 : Inport  Port=6  OutDataTypeStr=fixdt(0,1,0)  LockScale=on
  X7 : Inport  Port=7  OutDataTypeStr=fixdt(0,1,0)  LockScale=on
  X8 : Inport  Port=8  OutDataTypeStr=fixdt(0,1,0)  LockScale=on
  X9 : Inport  Port=9  OutDataTypeStr=fixdt(0,1,0)  LockScale=on
  X10 : Inport  Port=10  OutDataTypeStr=fixdt(0,1,0)  LockScale=on
  X11 : Inport  Port=11  OutDataTypeStr=fixdt(0,1,0)  LockScale=on
  X12 : Inport  Port=12  OutDataTypeStr=fixdt(0,1,0)  LockScale=on
  X13 : Inport  Port=13  OutDataTypeStr=fixdt(0,1,0)  LockScale=on
  X14 : Inport  Port=14  OutDataTypeStr=fixdt(0,1,0)  LockScale=on
  X15 : Inport  Port=15  OutDataTypeStr=fixdt(0,1,0)  LockScale=on
  Y : Inport  Port=16  LockScale=on
  N : Inport  Port=17  LockScale=on
  shifted_coeff : Inport  Port=18  LockScale=on
  EN_X : Inport  Port=19  OutDataTypeStr=fixdt(0,1,0)  LockScale=on
  Add : Sum  Inputs=++++++++++++++++
  Add2 : Sum  Inputs=+-
  Constant : Constant  Value=2
  Constant1 : Constant  Value=4
  Constant15 : Constant  Value=128
  Constant16 : Constant  Value=256
  Constant17 : Constant  Value=512
  Constant18 : Constant  Value=1024
  Constant19 : Constant  Value=2048
  Constant2 : Constant  Value=8
  Constant20 : Constant  Value=4096
  Constant21 : Constant  Value=8192
  Constant22 : Constant  Value=16384
  Constant28 : Constant  Value=32768
  Constant3 : Constant  Value=16
  Constant4 : Constant  Value=32
  Constant6 : Constant
  Constant8 : Constant  Value=64
  NOT : Logic  Operator=NOT  IconShape=distinctive  AllPortsSameDT=off  OutDataTypeStr=boolean
  Product{,1..6,8,16..23,28,142} (18 alike) : Product
  Switch_2 : Switch  Criteria=u2 ~= 0  OutDataTypeStr=fixdt(0,1,0)  SaturateOnIntegerOverflow=off  InputSameDT=off
  E_X : Outport  LockScale=on
  wires:
  Constant/1 -> Product/2
  X1/1 -> Product/1
  Constant1/1 -> Product1/2
  X2/1 -> Product1/1
  Constant2/1 -> Product2/2
  X3/1 -> Product2/1
  Constant6/1 -> Add/1
  Product/1 -> Add/2
  Product1/1 -> Add/3
  Product2/1 -> Add/4
  Add/1 -> Product6/1
  Add2/1 -> Product8/2, Product8/1
  Product4/1 -> Add/6
  Constant4/1 -> Product4/2
  Constant8/1 -> Product5/2
  X6/1 -> Product5/1
  Product3/1 -> Add/5
  X4/1 -> Product3/1
  Product5/1 -> Add/7
  X5/1 -> Product4/1
  Constant3/1 -> Product3/2
  Product19/1 -> Add/11
  Constant20/1 -> Product21/2
  Constant18/1 -> Product19/2
  Product18/1 -> Add/10
  Constant15/1 -> Product16/2
  Constant16/1 -> Product17/2
  X11/1 -> Product20/1
  Product20/1 -> Add/12
  X8/1 -> Product17/1
  X10/1 -> Product19/1
  Switch_2/1 -> Product16/1
  Constant19/1 -> Product20/2
  Product16/1 -> Add/8
  X9/1 -> Product18/1
  Constant17/1 -> Product18/2
  Product21/1 -> Add/13
  X12/1 -> Product21/1
  Product17/1 -> Add/9
  X14/1 -> Product23/1
  X15/1 -> Product28/1
  Constant28/1 -> Product28/2
  Product28/1 -> Add/16
  Product22/1 -> Add/14
  Product23/1 -> Add/15
  Constant21/1 -> Product22/2
  Constant22/1 -> Product23/2
  [EN_X] -> Switch_2/2
  X7/1 -> NOT/1, Switch_2/3  "PBIT1"
  NOT/1 -> Switch_2/1
  X13/1 -> Product22/1
  EN_X/1 -> [EN_X]
  shifted_coeff/1 -> [shifted_coeff]
  Product142/1 -> E_X/1
  [shifted_coeff] -> Product142/2
  Product6/1 -> Add2/1
  Product8/1 -> Product142/1
  N/1 -> Add2/2
  Y/1 -> Product6/2

== system Model_with_decision/X8 ==
  X1 : Inport  OutDataTypeStr=fixdt(0,1,0)  LockScale=on
  X2 : Inport  Port=2  OutDataTypeStr=fixdt(0,1,0)  LockScale=on
  X3 : Inport  Port=3  OutDataTypeStr=fixdt(0,1,0)  LockScale=on
  X4 : Inport  Port=4  OutDataTypeStr=fixdt(0,1,0)  LockScale=on
  X5 : Inport  Port=5  OutDataTypeStr=fixdt(0,1,0)  LockScale=on
  X6 : Inport  Port=6  OutDataTypeStr=fixdt(0,1,0)  LockScale=on
  X7 : Inport  Port=7  OutDataTypeStr=fixdt(0,1,0)  LockScale=on
  X8 : Inport  Port=8  OutDataTypeStr=fixdt(0,1,0)  LockScale=on
  X9 : Inport  Port=9  OutDataTypeStr=fixdt(0,1,0)  LockScale=on
  X10 : Inport  Port=10  OutDataTypeStr=fixdt(0,1,0)  LockScale=on
  X11 : Inport  Port=11  OutDataTypeStr=fixdt(0,1,0)  LockScale=on
  X12 : Inport  Port=12  OutDataTypeStr=fixdt(0,1,0)  LockScale=on
  X13 : Inport  Port=13  OutDataTypeStr=fixdt(0,1,0)  LockScale=on
  X14 : Inport  Port=14  OutDataTypeStr=fixdt(0,1,0)  LockScale=on
  X15 : Inport  Port=15  OutDataTypeStr=fixdt(0,1,0)  LockScale=on
  Y : Inport  Port=16  LockScale=on
  N : Inport  Port=17  LockScale=on
  shifted_coeff : Inport  Port=18  LockScale=on
  EN_X : Inport  Port=19  OutDataTypeStr=fixdt(0,1,0)  LockScale=on
  Add : Sum  Inputs=++++++++++++++++
  Add2 : Sum  Inputs=+-
  Constant : Constant  Value=2
  Constant1 : Constant  Value=4
  Constant15 : Constant  Value=128
  Constant16 : Constant  Value=256
  Constant17 : Constant  Value=512
  Constant18 : Constant  Value=1024
  Constant19 : Constant  Value=2048
  Constant2 : Constant  Value=8
  Constant20 : Constant  Value=4096
  Constant21 : Constant  Value=8192
  Constant22 : Constant  Value=16384
  Constant28 : Constant  Value=32768
  Constant3 : Constant  Value=16
  Constant4 : Constant  Value=32
  Constant6 : Constant
  Constant8 : Constant  Value=64
  NOT : Logic  Operator=NOT  IconShape=distinctive  AllPortsSameDT=off  OutDataTypeStr=boolean
  Product{,1..6,8,16..23,28,142} (18 alike) : Product
  Switch_2 : Switch  Criteria=u2 ~= 0  OutDataTypeStr=fixdt(0,1,0)  SaturateOnIntegerOverflow=off  InputSameDT=off
  E_X : Outport  LockScale=on
  wires:
  Constant/1 -> Product/2
  X1/1 -> Product/1
  Constant1/1 -> Product1/2
  X2/1 -> Product1/1
  Constant2/1 -> Product2/2
  X3/1 -> Product2/1
  Constant6/1 -> Add/1
  Product/1 -> Add/2
  Product1/1 -> Add/3
  Product2/1 -> Add/4
  Add/1 -> Product6/1
  Add2/1 -> Product8/2, Product8/1
  Product4/1 -> Add/6
  Constant4/1 -> Product4/2
  Constant8/1 -> Product5/2
  X6/1 -> Product5/1
  Product3/1 -> Add/5
  X4/1 -> Product3/1
  Product5/1 -> Add/7
  X5/1 -> Product4/1
  Constant3/1 -> Product3/2
  Product19/1 -> Add/11
  Constant20/1 -> Product21/2
  Constant18/1 -> Product19/2
  Product18/1 -> Add/10
  Constant15/1 -> Product16/2
  Constant16/1 -> Product17/2
  X11/1 -> Product20/1
  Product20/1 -> Add/12
  Switch_2/1 -> Product17/1
  X10/1 -> Product19/1
  X7/1 -> Product16/1
  Constant19/1 -> Product20/2
  Product16/1 -> Add/8
  X9/1 -> Product18/1
  Constant17/1 -> Product18/2
  Product21/1 -> Add/13
  X12/1 -> Product21/1
  Product17/1 -> Add/9
  X14/1 -> Product23/1
  X15/1 -> Product28/1
  Constant28/1 -> Product28/2
  Product28/1 -> Add/16
  Product22/1 -> Add/14
  Product23/1 -> Add/15
  Constant21/1 -> Product22/2
  Constant22/1 -> Product23/2
  [EN_X] -> Switch_2/2
  X8/1 -> Switch_2/3, NOT/1  "PBIT1"
  NOT/1 -> Switch_2/1
  X13/1 -> Product22/1
  EN_X/1 -> [EN_X]
  shifted_coeff/1 -> [shifted_coeff]
  Product142/1 -> E_X/1
  [shifted_coeff] -> Product142/2
  Product6/1 -> Add2/1
  Product8/1 -> Product142/1
  N/1 -> Add2/2
  Y/1 -> Product6/2

== system Model_with_decision/X9 ==
  X1 : Inport  OutDataTypeStr=fixdt(0,1,0)  LockScale=on
  X2 : Inport  Port=2  OutDataTypeStr=fixdt(0,1,0)  LockScale=on
  X3 : Inport  Port=3  OutDataTypeStr=fixdt(0,1,0)  LockScale=on
  X4 : Inport  Port=4  OutDataTypeStr=fixdt(0,1,0)  LockScale=on
  X5 : Inport  Port=5  OutDataTypeStr=fixdt(0,1,0)  LockScale=on
  X6 : Inport  Port=6  OutDataTypeStr=fixdt(0,1,0)  LockScale=on
  X7 : Inport  Port=7  OutDataTypeStr=fixdt(0,1,0)  LockScale=on
  X8 : Inport  Port=8  OutDataTypeStr=fixdt(0,1,0)  LockScale=on
  X9 : Inport  Port=9  OutDataTypeStr=fixdt(0,1,0)  LockScale=on
  X10 : Inport  Port=10  OutDataTypeStr=fixdt(0,1,0)  LockScale=on
  X11 : Inport  Port=11  OutDataTypeStr=fixdt(0,1,0)  LockScale=on
  X12 : Inport  Port=12  OutDataTypeStr=fixdt(0,1,0)  LockScale=on
  X13 : Inport  Port=13  OutDataTypeStr=fixdt(0,1,0)  LockScale=on
  X14 : Inport  Port=14  OutDataTypeStr=fixdt(0,1,0)  LockScale=on
  X15 : Inport  Port=15  OutDataTypeStr=fixdt(0,1,0)  LockScale=on
  Y : Inport  Port=16  LockScale=on
  N : Inport  Port=17  LockScale=on
  shifted_coeff : Inport  Port=18  LockScale=on
  EN_X : Inport  Port=19  OutDataTypeStr=fixdt(0,1,0)  LockScale=on
  Add : Sum  Inputs=++++++++++++++++
  Add2 : Sum  Inputs=+-
  Constant : Constant  Value=2
  Constant1 : Constant  Value=4
  Constant15 : Constant  Value=128
  Constant16 : Constant  Value=256
  Constant17 : Constant  Value=512
  Constant18 : Constant  Value=1024
  Constant19 : Constant  Value=2048
  Constant2 : Constant  Value=8
  Constant20 : Constant  Value=4096
  Constant21 : Constant  Value=8192
  Constant22 : Constant  Value=16384
  Constant28 : Constant  Value=32768
  Constant3 : Constant  Value=16
  Constant4 : Constant  Value=32
  Constant6 : Constant
  Constant8 : Constant  Value=64
  NOT : Logic  Operator=NOT  IconShape=distinctive  AllPortsSameDT=off  OutDataTypeStr=boolean
  Product{,1..6,8,16..23,28,142} (18 alike) : Product
  Switch_2 : Switch  Criteria=u2 ~= 0  OutDataTypeStr=fixdt(0,1,0)  SaturateOnIntegerOverflow=off  InputSameDT=off
  E_X : Outport  LockScale=on
  wires:
  Y/1 -> Product6/2
  N/1 -> Add2/2
  Product8/1 -> Product142/1
  Product6/1 -> Add2/1
  [SCALE] -> Product142/2
  Product142/1 -> E_X/1
  shifted_coeff/1 -> [shifted_coeff]
  EN_X/1 -> [EN_X]
  X13/1 -> Product22/1
  NOT/1 -> Switch_2/1
  X9/1 -> Switch_2/3, NOT/1  "PBIT1"
  [EN_X] -> Switch_2/2
  Constant22/1 -> Product23/2
  Constant21/1 -> Product22/2
  Product23/1 -> Add/15
  Product22/1 -> Add/14
  Product28/1 -> Add/16
  Constant28/1 -> Product28/2
  X15/1 -> Product28/1
  X14/1 -> Product23/1
  Product17/1 -> Add/9
  X12/1 -> Product21/1
  Product21/1 -> Add/13
  Constant17/1 -> Product18/2
  Switch_2/1 -> Product18/1
  Product16/1 -> Add/8
  Constant19/1 -> Product20/2
  X7/1 -> Product16/1
  X10/1 -> Product19/1
  X8/1 -> Product17/1
  Product20/1 -> Add/12
  X11/1 -> Product20/1
  Constant16/1 -> Product17/2
  Constant15/1 -> Product16/2
  Product18/1 -> Add/10
  Constant18/1 -> Product19/2
  Constant20/1 -> Product21/2
  Product19/1 -> Add/11
  Constant3/1 -> Product3/2
  X5/1 -> Product4/1
  Product5/1 -> Add/7
  X4/1 -> Product3/1
  Product3/1 -> Add/5
  X6/1 -> Product5/1
  Constant8/1 -> Product5/2
  Constant4/1 -> Product4/2
  Product4/1 -> Add/6
  Add2/1 -> Product8/1, Product8/2
  Add/1 -> Product6/1
  Product2/1 -> Add/4
  Product1/1 -> Add/3
  Product/1 -> Add/2
  Constant6/1 -> Add/1
  X3/1 -> Product2/1
  Constant2/1 -> Product2/2
  X2/1 -> Product1/1
  Constant1/1 -> Product1/2
  X1/1 -> Product/1
  Constant/1 -> Product/2

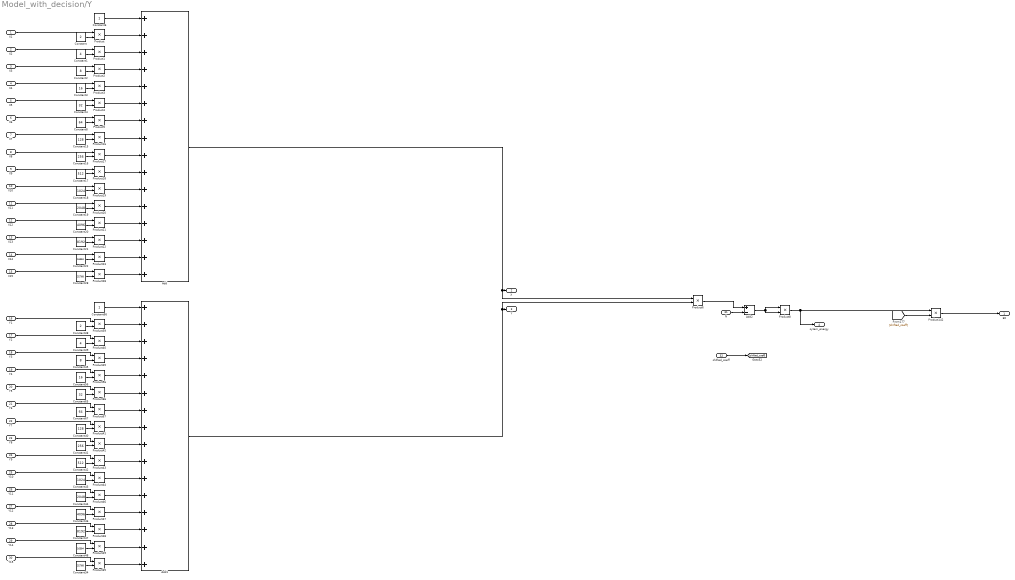
== system Model_with_decision/Y ==
  X1 : Inport  OutDataTypeStr=fixdt(0,1,0)  LockScale=on
  X2 : Inport  Port=2  OutDataTypeStr=fixdt(0,1,0)  LockScale=on
  X3 : Inport  Port=3  OutDataTypeStr=fixdt(0,1,0)  LockScale=on
  X4 : Inport  Port=4  OutDataTypeStr=fixdt(0,1,0)  LockScale=on
  X5 : Inport  Port=5  OutDataTypeStr=fixdt(0,1,0)  LockScale=on
  X6 : Inport  Port=6  OutDataTypeStr=fixdt(0,1,0)  LockScale=on
  X7 : Inport  Port=7  OutDataTypeStr=fixdt(0,1,0)  LockScale=on
  X8 : Inport  Port=8  OutDataTypeStr=fixdt(0,1,0)  LockScale=on
  X9 : Inport  Port=9  OutDataTypeStr=fixdt(0,1,0)  LockScale=on
  X10 : Inport  Port=10  OutDataTypeStr=fixdt(0,1,0)  LockScale=on
  X11 : Inport  Port=11  OutDataTypeStr=fixdt(0,1,0)  LockScale=on
  X12 : Inport  Port=12  OutDataTypeStr=fixdt(0,1,0)  LockScale=on
  X13 : Inport  Port=13  OutDataTypeStr=fixdt(0,1,0)  LockScale=on
  X14 : Inport  Port=14  OutDataTypeStr=fixdt(0,1,0)  LockScale=on
  X15 : Inport  Port=15  OutDataTypeStr=fixdt(0,1,0)  LockScale=on
  Y1 : Inport  Port=16  OutDataTypeStr=fixdt(0,1,0)  LockScale=on
  Y2 : Inport  Port=17  OutDataTypeStr=fixdt(0,1,0)  LockScale=on
  Y3 : Inport  Port=18  OutDataTypeStr=fixdt(0,1,0)  LockScale=on
  Y4 : Inport  Port=19  OutDataTypeStr=fixdt(0,1,0)  LockScale=on
  Y5 : Inport  Port=20  OutDataTypeStr=fixdt(0,1,0)  LockScale=on
  Y6 : Inport  Port=21  OutDataTypeStr=fixdt(0,1,0)  LockScale=on
  Y7 : Inport  Port=22  OutDataTypeStr=fixdt(0,1,0)  LockScale=on
  Y8 : Inport  Port=23  OutDataTypeStr=fixdt(0,1,0)  LockScale=on
  Y9 : Inport  Port=24  OutDataTypeStr=fixdt(0,1,0)  LockScale=on
  Y10 : Inport  Port=25  OutDataTypeStr=fixdt(0,1,0)  LockScale=on
  Y11 : Inport  Port=26  OutDataTypeStr=fixdt(0,1,0)  LockScale=on
  Y12 : Inport  Port=27  OutDataTypeStr=fixdt(0,1,0)  LockScale=on
  Y13 : Inport  Port=28  OutDataTypeStr=fixdt(0,1,0)  LockScale=on
  Y14 : Inport  Port=29  OutDataTypeStr=fixdt(0,1,0)  LockScale=on
  Y15 : Inport  Port=30  OutDataTypeStr=fixdt(0,1,0)  LockScale=on
  N : Inport  Port=31  LockScale=on
  shifted_coeff : Inport  Port=32  LockScale=on
  Add : Sum  Inputs=++++++++++++++++
  Add1 : Sum  Inputs=++++++++++++++++
  Add2 : Sum  Inputs=+-
  Constant : Constant  Value=2
  Constant1 : Constant  Value=4
  Constant15 : Constant  Value=128
  Constant16 : Constant  Value=256
  Constant17 : Constant  Value=512
  Constant18 : Constant  Value=1024
  Constant19 : Constant  Value=2048
  Constant2 : Constant  Value=8
  Constant20 : Constant  Value=4096
  Constant21 : Constant  Value=8192
  Constant22 : Constant  Value=16384
  Constant28 : Constant  Value=32768
  Constant3 : Constant  Value=16
  Constant34 : Constant  Value=32768
  Constant38 : Constant  Value=2
  Constant39 : Constant  Value=4
  Constant4 : Constant  Value=32
  Constant40 : Constant  Value=128
  Constant41 : Constant  Value=256
  Constant42 : Constant  Value=512
  Constant43 : Constant  Value=1024
  Constant44 : Constant  Value=2048
  Constant45 : Constant  Value=8
  Constant46 : Constant  Value=4096
  Constant47 : Constant  Value=8192
  Constant48 : Constant  Value=16384
  Constant56 : Constant  Value=16
  Constant6 : Constant
  Constant65 : Constant  Value=32
  Constant66 : Constant
  Constant67 : Constant  Value=64
  Constant8 : Constant  Value=64
  Product{,1..6,8,16..23,28,35,39..49,56,66..67,142} (33 alike) : Product
  E0 : Outport  LockScale=on
  X : Outport  Port=2  LockScale=on
  Y : Outport  Port=3  LockScale=on
  sytem_energy : Outport  Port=4  LockScale=on
  wires:
  Constant/1 -> Product/2
  X1/1 -> Product/1
  Constant1/1 -> Product1/2
  X2/1 -> Product1/1
  Constant2/1 -> Product2/2
  X3/1 -> Product2/1
  Constant6/1 -> Add/1
  Product/1 -> Add/2
  Product1/1 -> Add/3
  Product2/1 -> Add/4
  Add/1 -> Product6/1, X/1
  Add2/1 -> Product8/2, Product8/1
  Product4/1 -> Add/6
  Constant4/1 -> Product4/2
  Constant8/1 -> Product5/2
  X6/1 -> Product5/1
  Product3/1 -> Add/5
  X4/1 -> Product3/1
  Product5/1 -> Add/7
  X5/1 -> Product4/1
  Constant3/1 -> Product3/2
  Product19/1 -> Add/11
  Constant20/1 -> Product21/2
  Constant18/1 -> Product19/2
  Product18/1 -> Add/10
  Constant15/1 -> Product16/2
  Constant16/1 -> Product17/2
  X11/1 -> Product20/1
  Product20/1 -> Add/12
  X8/1 -> Product17/1
  X10/1 -> Product19/1
  X7/1 -> Product16/1
  Constant19/1 -> Product20/2
  Product16/1 -> Add/8
  X9/1 -> Product18/1
  Constant17/1 -> Product18/2
  Product21/1 -> Add/13
  X12/1 -> Product21/1
  Product17/1 -> Add/9
  X14/1 -> Product23/1
  X15/1 -> Product28/1
  Constant28/1 -> Product28/2
  Product28/1 -> Add/16
  Product22/1 -> Add/14
  Product23/1 -> Add/15
  Constant21/1 -> Product22/2
  Constant22/1 -> Product23/2
  Constant43/1 -> Product44/2
  Product56/1 -> Add1/5
  Constant44/1 -> Product46/2
  Constant38/1 -> Product39/2
  Product47/1 -> Add1/13
  Product67/1 -> Add1/7
  Product40/1 -> Add1/3
  Product43/1 -> Add1/10
  Product66/1 -> Add1/6
  Product41/1 -> Add1/8
  Constant48/1 -> Product49/2
  Constant41/1 -> Product42/2
  Product45/1 -> Add1/4
  Product49/1 -> Add1/15
  Constant40/1 -> Product41/2
  Constant45/1 -> Product45/2
  Product48/1 -> Add1/14
  Constant65/1 -> Product66/2
  Product42/1 -> Add1/9
  Constant42/1 -> Product43/2
  Constant56/1 -> Product56/2
  Product39/1 -> Add1/2
  Constant66/1 -> Add1/1
  Constant46/1 -> Product47/2
  Constant67/1 -> Product67/2
  Product46/1 -> Add1/12
  Product44/1 -> Add1/11
  Constant47/1 -> Product48/2
  Constant39/1 -> Product40/2
  Add1/1 -> Product6/2, Y/1
  X13/1 -> Product22/1
  shifted_coeff/1 -> [shifted_coeff]
  Product142/1 -> E0/1
  [shifted_coeff] -> Product142/2
  Product6/1 -> Add2/1
  N/1 -> Add2/2
  Y1/1 -> Product39/1
  Y2/1 -> Product40/1
  Y3/1 -> Product45/1
  Y4/1 -> Product56/1
  Y5/1 -> Product66/1
  Y6/1 -> Product67/1
  Y7/1 -> Product41/1
  Y8/1 -> Product42/1
  Y9/1 -> Product43/1
  Y10/1 -> Product44/1
  Y11/1 -> Product46/1
  Y12/1 -> Product47/1
  Y13/1 -> Product48/1
  Y14/1 -> Product49/1
  Product8/1 -> sytem_energy/1, Product142/1
  Product35/1 -> Add1/16
  Constant34/1 -> Product35/2
  Y15/1 -> Product35/1

== system Model_with_decision/Y1 ==
  Y1 : Inport  OutDataTypeStr=fixdt(0,1,0)  LockScale=on
  Y2 : Inport  Port=2  OutDataTypeStr=fixdt(0,1,0)  LockScale=on
  Y3 : Inport  Port=3  OutDataTypeStr=fixdt(0,1,0)  LockScale=on
  Y4 : Inport  Port=4  OutDataTypeStr=fixdt(0,1,0)  LockScale=on
  Y5 : Inport  Port=5  OutDataTypeStr=fixdt(0,1,0)  LockScale=on
  Y6 : Inport  Port=6  OutDataTypeStr=fixdt(0,1,0)  LockScale=on
  Y7 : Inport  Port=7  OutDataTypeStr=fixdt(0,1,0)  LockScale=on
  Y8 : Inport  Port=8  OutDataTypeStr=fixdt(0,1,0)  LockScale=on
  Y9 : Inport  Port=9  OutDataTypeStr=fixdt(0,1,0)  LockScale=on
  Y10 : Inport  Port=10  OutDataTypeStr=fixdt(0,1,0)  LockScale=on
  Y11 : Inport  Port=11  OutDataTypeStr=fixdt(0,1,0)  LockScale=on
  Y12 : Inport  Port=12  OutDataTypeStr=fixdt(0,1,0)  LockScale=on
  Y13 : Inport  Port=13  OutDataTypeStr=fixdt(0,1,0)  LockScale=on
  Y14 : Inport  Port=14  OutDataTypeStr=fixdt(0,1,0)  LockScale=on
  Y15 : Inport  Port=15  OutDataTypeStr=fixdt(0,1,0)  LockScale=on
  X : Inport  Port=16
  N : Inport  Port=17  LockScale=on
  shifted_coeff : Inport  Port=18  LockScale=on
  EN_Y : Inport  Port=19  OutDataTypeStr=fixdt(0,1,0)  LockScale=on
  Add : Sum  Inputs=++++++++++++++++
  Add2 : Sum  Inputs=+-
  Constant : Constant  Value=2
  Constant1 : Constant  Value=4
  Constant15 : Constant  Value=128
  Constant16 : Constant  Value=256
  Constant17 : Constant  Value=512
  Constant18 : Constant  Value=1024
  Constant19 : Constant  Value=2048
  Constant2 : Constant  Value=8
  Constant20 : Constant  Value=4096
  Constant21 : Constant  Value=8192
  Constant22 : Constant  Value=16384
  Constant3 : Constant  Value=16
  Constant34 : Constant  Value=32768
  Constant4 : Constant  Value=32
  Constant6 : Constant
  Constant8 : Constant  Value=64
  NOT : Logic  Operator=NOT  IconShape=distinctive  AllPortsSameDT=off  OutDataTypeStr=boolean
  Product{,1..6,8,16..23,35,142} (18 alike) : Product
  Switch_2 : Switch  Criteria=u2 ~= 0  OutDataTypeStr=fixdt(0,1,0)  SaturateOnIntegerOverflow=off  InputSameDT=off
  E_Y : Outport  LockScale=on
  wires:
  Constant/1 -> Product/2
  Switch_2/1 -> Product/1
  Constant1/1 -> Product1/2
  Y2/1 -> Product1/1
  Constant2/1 -> Product2/2
  Y3/1 -> Product2/1
  Constant6/1 -> Add/1
  Product/1 -> Add/2
  Product1/1 -> Add/3
  Product2/1 -> Add/4
  Add/1 -> Product6/1
  Add2/1 -> Product8/2, Product8/1
  Product4/1 -> Add/6
  Constant4/1 -> Product4/2
  Constant8/1 -> Product5/2
  Y6/1 -> Product5/1
  Product3/1 -> Add/5
  Y4/1 -> Product3/1
  Product5/1 -> Add/7
  Y5/1 -> Product4/1
  Constant3/1 -> Product3/2
  Product19/1 -> Add/11
  Constant20/1 -> Product21/2
  Constant18/1 -> Product19/2
  Product18/1 -> Add/10
  Constant15/1 -> Product16/2
  Constant16/1 -> Product17/2
  Y11/1 -> Product20/1
  Product20/1 -> Add/12
  Y8/1 -> Product17/1
  Y10/1 -> Product19/1
  Y7/1 -> Product16/1
  Constant19/1 -> Product20/2
  Product16/1 -> Add/8
  Y9/1 -> Product18/1
  Constant17/1 -> Product18/2
  Product21/1 -> Add/13
  Y12/1 -> Product21/1
  Product17/1 -> Add/9
  Y14/1 -> Product23/1
  Product22/1 -> Add/14
  Product23/1 -> Add/15
  Constant21/1 -> Product22/2
  Constant22/1 -> Product23/2
  [EN_Y] -> Switch_2/2
  Y1/1 -> NOT/1, Switch_2/3  "PBIT28"
  NOT/1 -> Switch_2/1
  Y13/1 -> Product22/1
  EN_Y/1 -> [EN_Y]
  shifted_coeff/1 -> [shifted_coeff]
  Product142/1 -> E_Y/1
  [shifted_coeff] -> Product142/2
  Product6/1 -> Add2/1
  Product8/1 -> Product142/1
  N/1 -> Add2/2
  X/1 -> Product6/2
  Y15/1 -> Product35/1
  Product35/1 -> Add/16
  Constant34/1 -> Product35/2

== system Model_with_decision/Y10 ==
  Y1 : Inport  OutDataTypeStr=fixdt(0,1,0)  LockScale=on
  Y2 : Inport  Port=2  OutDataTypeStr=fixdt(0,1,0)  LockScale=on
  Y3 : Inport  Port=3  OutDataTypeStr=fixdt(0,1,0)  LockScale=on
  Y4 : Inport  Port=4  OutDataTypeStr=fixdt(0,1,0)  LockScale=on
  Y5 : Inport  Port=5  OutDataTypeStr=fixdt(0,1,0)  LockScale=on
  Y6 : Inport  Port=6  OutDataTypeStr=fixdt(0,1,0)  LockScale=on
  Y7 : Inport  Port=7  OutDataTypeStr=fixdt(0,1,0)  LockScale=on
  Y8 : Inport  Port=8  OutDataTypeStr=fixdt(0,1,0)  LockScale=on
  Y9 : Inport  Port=9  OutDataTypeStr=fixdt(0,1,0)  LockScale=on
  Y10 : Inport  Port=10  OutDataTypeStr=fixdt(0,1,0)  LockScale=on
  Y11 : Inport  Port=11  OutDataTypeStr=fixdt(0,1,0)  LockScale=on
  Y12 : Inport  Port=12  OutDataTypeStr=fixdt(0,1,0)  LockScale=on
  Y13 : Inport  Port=13  OutDataTypeStr=fixdt(0,1,0)  LockScale=on
  Y14 : Inport  Port=14  OutDataTypeStr=fixdt(0,1,0)  LockScale=on
  Y15 : Inport  Port=15  OutDataTypeStr=fixdt(0,1,0)  LockScale=on
  X : Inport  Port=16
  N : Inport  Port=17  LockScale=on
  shifted_coeff : Inport  Port=18  LockScale=on
  EN_Y : Inport  Port=19  OutDataTypeStr=fixdt(0,1,0)  LockScale=on
  Add : Sum  Inputs=++++++++++++++++
  Add2 : Sum  Inputs=+-
  Constant : Constant  Value=2
  Constant1 : Constant  Value=4
  Constant15 : Constant  Value=128
  Constant16 : Constant  Value=256
  Constant17 : Constant  Value=512
  Constant18 : Constant  Value=1024
  Constant19 : Constant  Value=2048
  Constant2 : Constant  Value=8
  Constant20 : Constant  Value=4096
  Constant21 : Constant  Value=8192
  Constant22 : Constant  Value=16384
  Constant3 : Constant  Value=16
  Constant34 : Constant  Value=32768
  Constant4 : Constant  Value=32
  Constant6 : Constant
  Constant8 : Constant  Value=64
  NOT : Logic  Operator=NOT  IconShape=distinctive  AllPortsSameDT=off  OutDataTypeStr=boolean
  Product{,1..6,8,16..23,35,142} (18 alike) : Product
  Switch_2 : Switch  Criteria=u2 ~= 0  OutDataTypeStr=fixdt(0,1,0)  SaturateOnIntegerOverflow=off  InputSameDT=off
  E_Y : Outport  LockScale=on
  wires:
  Constant34/1 -> Product35/2
  Product35/1 -> Add/16
  Y15/1 -> Product35/1
  X/1 -> Product6/2
  N/1 -> Add2/2
  Product8/1 -> Product142/1
  Product6/1 -> Add2/1
  [shifted_coeff] -> Product142/2
  Product142/1 -> E_Y/1
  shifted_coeff/1 -> [shifted_coeff]
  EN_Y/1 -> [EN_Y]
  Y13/1 -> Product22/1
  NOT/1 -> Switch_2/1
  Y10/1 -> Switch_2/3, NOT/1  "PBIT28"
  [EN_Y] -> Switch_2/2
  Constant22/1 -> Product23/2
  Constant21/1 -> Product22/2
  Product23/1 -> Add/15
  Product22/1 -> Add/14
  Y14/1 -> Product23/1
  Product17/1 -> Add/9
  Y12/1 -> Product21/1
  Product21/1 -> Add/13
  Constant17/1 -> Product18/2
  Y9/1 -> Product18/1
  Product16/1 -> Add/8
  Constant19/1 -> Product20/2
  Y7/1 -> Product16/1
  Switch_2/1 -> Product19/1
  Y8/1 -> Product17/1
  Product20/1 -> Add/12
  Y11/1 -> Product20/1
  Constant16/1 -> Product17/2
  Constant15/1 -> Product16/2
  Product18/1 -> Add/10
  Constant18/1 -> Product19/2
  Constant20/1 -> Product21/2
  Product19/1 -> Add/11
  Constant3/1 -> Product3/2
  Y5/1 -> Product4/1
  Product5/1 -> Add/7
  Y4/1 -> Product3/1
  Product3/1 -> Add/5
  Y6/1 -> Product5/1
  Constant8/1 -> Product5/2
  Constant4/1 -> Product4/2
  Product4/1 -> Add/6
  Add2/1 -> Product8/1, Product8/2
  Add/1 -> Product6/1
  Product2/1 -> Add/4
  Product1/1 -> Add/3
  Product/1 -> Add/2
  Constant6/1 -> Add/1
  Y3/1 -> Product2/1
  Constant2/1 -> Product2/2
  Y2/1 -> Product1/1
  Constant1/1 -> Product1/2
  Y1/1 -> Product/1
  Constant/1 -> Product/2

== system Model_with_decision/Y11 ==
  Y1 : Inport  OutDataTypeStr=fixdt(0,1,0)  LockScale=on
  Y2 : Inport  Port=2  OutDataTypeStr=fixdt(0,1,0)  LockScale=on
  Y3 : Inport  Port=3  OutDataTypeStr=fixdt(0,1,0)  LockScale=on
  Y4 : Inport  Port=4  OutDataTypeStr=fixdt(0,1,0)  LockScale=on
  Y5 : Inport  Port=5  OutDataTypeStr=fixdt(0,1,0)  LockScale=on
  Y6 : Inport  Port=6  OutDataTypeStr=fixdt(0,1,0)  LockScale=on
  Y7 : Inport  Port=7  OutDataTypeStr=fixdt(0,1,0)  LockScale=on
  Y8 : Inport  Port=8  OutDataTypeStr=fixdt(0,1,0)  LockScale=on
  Y9 : Inport  Port=9  OutDataTypeStr=fixdt(0,1,0)  LockScale=on
  Y10 : Inport  Port=10  OutDataTypeStr=fixdt(0,1,0)  LockScale=on
  Y11 : Inport  Port=11  OutDataTypeStr=fixdt(0,1,0)  LockScale=on
  Y12 : Inport  Port=12  OutDataTypeStr=fixdt(0,1,0)  LockScale=on
  Y13 : Inport  Port=13  OutDataTypeStr=fixdt(0,1,0)  LockScale=on
  Y14 : Inport  Port=14  OutDataTypeStr=fixdt(0,1,0)  LockScale=on
  Y15 : Inport  Port=15  OutDataTypeStr=fixdt(0,1,0)  LockScale=on
  X : Inport  Port=16
  N : Inport  Port=17  LockScale=on
  shifted_coeff : Inport  Port=18  LockScale=on
  EN_Y : Inport  Port=19  OutDataTypeStr=fixdt(0,1,0)  LockScale=on
  Add : Sum  Inputs=++++++++++++++++
  Add2 : Sum  Inputs=+-
  Constant : Constant  Value=2
  Constant1 : Constant  Value=4
  Constant15 : Constant  Value=128
  Constant16 : Constant  Value=256
  Constant17 : Constant  Value=512
  Constant18 : Constant  Value=1024
  Constant19 : Constant  Value=2048
  Constant2 : Constant  Value=8
  Constant20 : Constant  Value=4096
  Constant21 : Constant  Value=8192
  Constant22 : Constant  Value=16384
  Constant3 : Constant  Value=16
  Constant34 : Constant  Value=32768
  Constant4 : Constant  Value=32
  Constant6 : Constant
  Constant8 : Constant  Value=64
  NOT : Logic  Operator=NOT  IconShape=distinctive  AllPortsSameDT=off  OutDataTypeStr=boolean
  Product{,1..6,8,16..23,35,142} (18 alike) : Product
  Switch_2 : Switch  Criteria=u2 ~= 0  OutDataTypeStr=fixdt(0,1,0)  SaturateOnIntegerOverflow=off  InputSameDT=off
  E_Y : Outport  LockScale=on
  wires:
  Constant34/1 -> Product35/2
  Product35/1 -> Add/16
  Y15/1 -> Product35/1
  X/1 -> Product6/2
  N/1 -> Add2/2
  Product8/1 -> Product142/1
  Product6/1 -> Add2/1
  [shifted_coeff] -> Product142/2
  Product142/1 -> E_Y/1
  shifted_coeff/1 -> [shifted_coeff]
  EN_Y/1 -> [EN_Y]
  Y13/1 -> Product22/1
  NOT/1 -> Switch_2/1
  Y11/1 -> NOT/1, Switch_2/3  "PBIT28"
  [EN_Y] -> Switch_2/2
  Constant22/1 -> Product23/2
  Constant21/1 -> Product22/2
  Product23/1 -> Add/15
  Product22/1 -> Add/14
  Y14/1 -> Product23/1
  Product17/1 -> Add/9
  Y12/1 -> Product21/1
  Product21/1 -> Add/13
  Constant17/1 -> Product18/2
  Y9/1 -> Product18/1
  Product16/1 -> Add/8
  Constant19/1 -> Product20/2
  Y7/1 -> Product16/1
  Y10/1 -> Product19/1
  Y8/1 -> Product17/1
  Product20/1 -> Add/12
  Switch_2/1 -> Product20/1
  Constant16/1 -> Product17/2
  Constant15/1 -> Product16/2
  Product18/1 -> Add/10
  Constant18/1 -> Product19/2
  Constant20/1 -> Product21/2
  Product19/1 -> Add/11
  Constant3/1 -> Product3/2
  Y5/1 -> Product4/1
  Product5/1 -> Add/7
  Y4/1 -> Product3/1
  Product3/1 -> Add/5
  Y6/1 -> Product5/1
  Constant8/1 -> Product5/2
  Constant4/1 -> Product4/2
  Product4/1 -> Add/6
  Add2/1 -> Product8/1, Product8/2
  Add/1 -> Product6/1
  Product2/1 -> Add/4
  Product1/1 -> Add/3
  Product/1 -> Add/2
  Constant6/1 -> Add/1
  Y3/1 -> Product2/1
  Constant2/1 -> Product2/2
  Y2/1 -> Product1/1
  Constant1/1 -> Product1/2
  Y1/1 -> Product/1
  Constant/1 -> Product/2
